simulink model "EnrouleurHG_Bode"  (R2024b)
settings: Solver=VariableStepAuto  StartTime=0.0  StopTime=1.2  RelTol=1e-3
values from neighbouring files (symbols this model uses):
  fv = 0    [parametres.m]
  Jm = 13.1/1000/10000    (= 1.31e-06)    [parametres.m]
  Kadapt = Kcapt/Rt    (= 52.1518917524)    [parametres.m]
  Kcapt = 8192/2/pi    (= 1303.79729381)    [parametres.m]
  Kcm = 25.5e-3    (= 0.0255)    [parametres.m]
  KCou_I = 900    [parametres.m]
  KCou_P = 2000    [parametres.m]
  KDSI = KPos_D*80/1000000    (= 0.0736)    [parametres.m]
  Kem = 1/(374 *2*pi/60)    (= 0.0255328785709)    [parametres.m]
  KPos_I = 270    [parametres.m]
  KPos_P = 215    [parametres.m]
  KPSI = KPos_P*10/1000    (= 2.15)    [parametres.m]
  Lm = 0.77e-3    (= 0.00077)    [parametres.m]
  r = 1/18    (= 0.0555555555556)    [parametres.m]
  Rm = 7.36    [parametres.m]
  Rt = 25    [parametres.m]
libraries: simulink x2, slctrl_linear x1
settings Model: Creator=xavier.pessoles2  LastModifiedBy=xpess

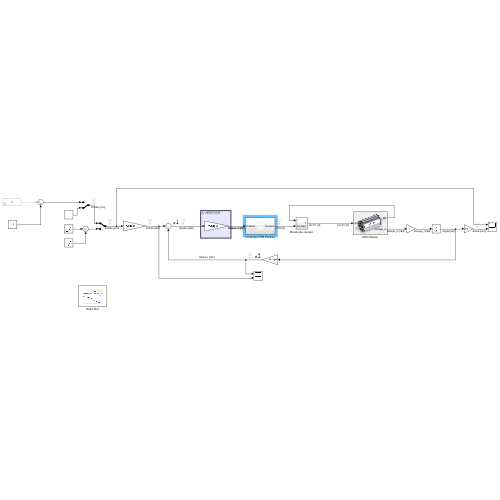
[thumbnail: Simulink's stored preview of the top-level diagram]
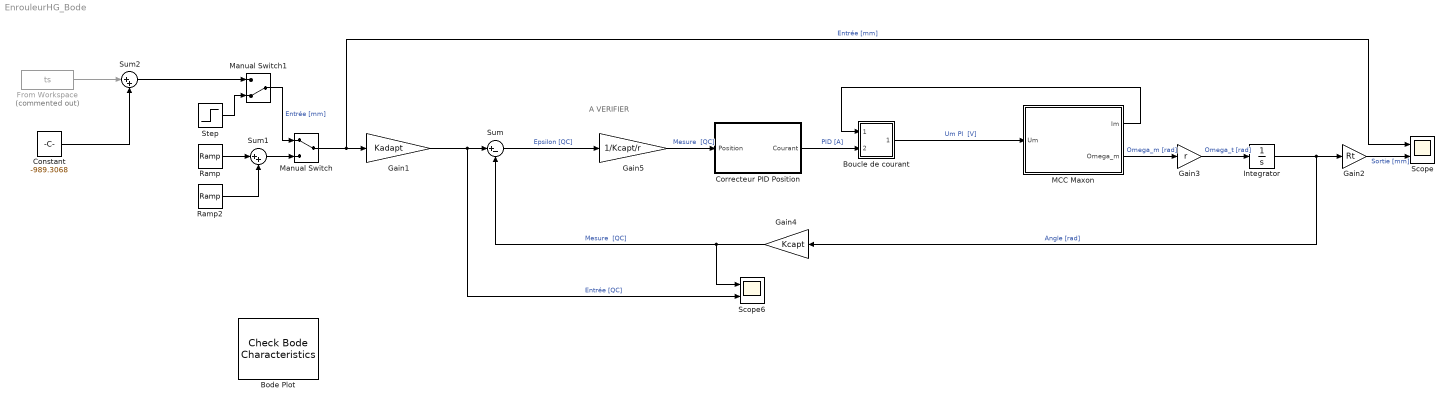
== system EnrouleurHG_Bode ==
  note: A VERIFIER
  Bode Plot : slctrl_linear/Check Bode  Characteristics  InstantiateOnLoad=on  SaveOperatingPoints=off  LinearizationIOs={'/Sum', 1, 'in', 'on', '';'/Gain4', 1, 'out', 'on', ''}  LinearizeAt=SnapshotTimes  SnapshotTimes=[0]  TriggerType=rising  SampleTime=auto  RateConversionMethod=zoh  PreWarpFreq=10  UseExactDelayModel=off  UseFullBlockNameLabels=off  UseBusSignalLabels=off  enabled=on  stopWhenAssertionFail=off  export=off  ViewDlgPos=[1 49 1280 599.333333333333]  OpenViewOnLoad=off  LaunchViewOnOpen=on  FrequencyUnits=rad/s  MagnitudeUnits=dB  PhaseUnits=deg  TimeUnits=seconds  EnableUpperBound=off  UpperBoundFrequencies=[]  UpperBoundMagnitudes=[]  EnableLowerBound=off  LowerBoundFrequencies=[]  LowerBoundMagnitudes=[]
      settings: LibrarySourceBlock=slctrlblks/Linear Analysis Plots/Bode Plot  SaveToWorkspace=off  SaveName=sys
  Boucle de courant : Subsystem
  Constant : Constant  Value=-989.3068
  Correcteur PID Position : Subsystem
  From Workspace : FromWorkspace  Commented=on  VariableName=ts
  Gain1 : Gain  Gain=Kadapt
  Gain2 : Gain  Gain=Rt
  Gain3 : Gain  Gain=r
  Gain4 : Gain  Gain=Kcapt
  Gain5 : Gain  Gain=1/Kcapt/r
  Integrator : Integrator
  MCC Maxon : Subsystem
      mask Display: image('MCC.png');
  Manual Switch : ManualSwitch
  Manual Switch1 : ManualSwitch  CurrentSetting=0
  Ramp : simulink/Sources/Ramp  slope=378  start=0  InitialOutput=0
  Ramp2 : simulink/Sources/Ramp  slope=-378  start=1  InitialOutput=0
  Scope : Scope  NumInputPorts=2
  Scope6 : Scope  NumInputPorts=2
  Step : Step  Time=0  After=0  SampleTime=0
  Sum : Sum  Inputs=|+-
  Sum1 : Sum  Inputs=|++
  Sum2 : Sum  Inputs=|++
  wires:
  Gain3/1 -> Integrator/1  "Omega_t [rad]"
  MCC Maxon/2(Omega_m) -> Gain3/1  "Omega_m [rad]"
  Sum/1 -> Gain5/1  "Epsilon [QC]"
  MCC Maxon/1(Im) -> Boucle de courant/1(In1)
  Boucle de courant/1(Out1) -> MCC Maxon/1(Um)  "Um PI  [V]"
  Gain4/1 -> Scope6/1, Sum/2  "Mesure  [QC]"
  Gain1/1 -> Sum/1, Scope6/2  "Entrée [QC]"
  Gain2/1 -> Scope/2  "Sortie [mm]"
  Integrator/1 -> Gain2/1, Gain4/1  "Angle [rad]"
  Ramp/1 -> Sum1/1
  Ramp2/1 -> Sum1/2
  Sum1/1 -> Manual Switch/2
  Manual Switch/1 -> Gain1/1, Scope/1  "Entrée [mm]"
  Gain5/1 -> Correcteur PID Position/1(Position)  "Mesure  [QC]"
  Manual Switch1/1 -> Manual Switch/1  "Entrée [mm]"
  Step/1 -> Manual Switch1/2
  From Workspace/1 -> Sum2/1
  Sum2/1 -> Manual Switch1/1
  Constant/1 -> Sum2/2
  Correcteur PID Position/1(Courant) -> Boucle de courant/2(Courant)  "PID [A]"

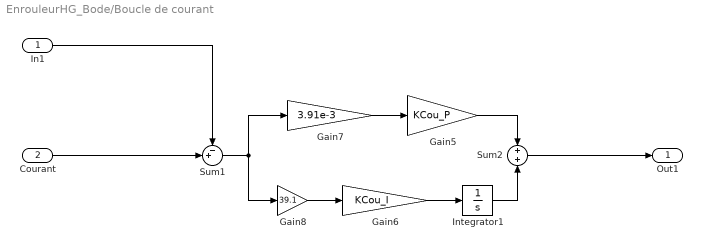
== system EnrouleurHG_Bode/Boucle de courant ==
  In1 : Inport
  Courant : Inport  Port=2
  Gain5 : Gain  Gain=KCou_P
  Gain6 : Gain  Gain=KCou_I
  Gain7 : Gain  Gain=3.91e-3
  Gain8 : Gain  Gain=39.1
  Integrator1 : Integrator
  Sum1 : Sum  Inputs=-+|
  Sum2 : Sum  Inputs=+|+
  Out1 : Outport
  wires:
  Sum1/1 -> Gain7/1, Gain8/1
  Gain5/1 -> Sum2/1
  Sum2/1 -> Out1/1
  Integrator1/1 -> Sum2/2
  Gain8/1 -> Gain6/1
  In1/1 -> Sum1/1
  Gain7/1 -> Gain5/1
  Gain6/1 -> Integrator1/1
  Courant/1 -> Sum1/2

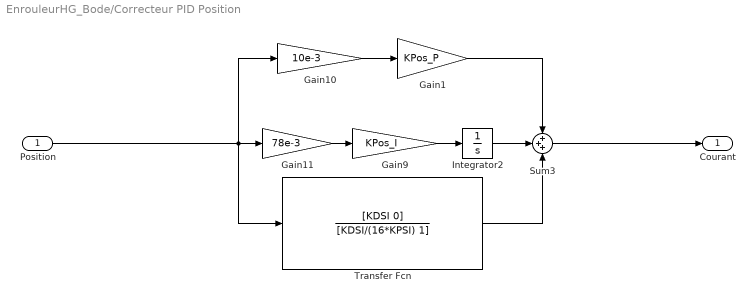
== system EnrouleurHG_Bode/Correcteur PID Position ==
  Position : Inport
  Gain1 : Gain  Gain=KPos_P
  Gain10 : Gain  Gain=10e-3
  Gain11 : Gain  Gain=78e-3
  Gain9 : Gain  Gain=KPos_I
  Integrator2 : Integrator
  Sum3 : Sum  Inputs=+++
  Transfer Fcn : TransferFcn  Numerator=[KDSI 0]  Denominator=[KDSI/(16*KPSI) 1]
  Courant : Outport
  wires:
  Gain1/1 -> Sum3/1
  Position/1 -> Gain10/1, Transfer Fcn/1, Gain11/1
  Gain9/1 -> Integrator2/1
  Sum3/1 -> Courant/1
  Integrator2/1 -> Sum3/2
  Gain10/1 -> Gain1/1
  Gain11/1 -> Gain9/1
  Transfer Fcn/1 -> Sum3/3

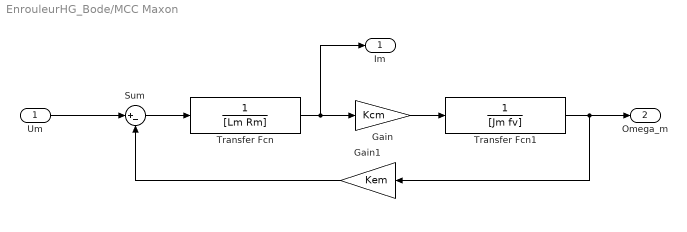
== system EnrouleurHG_Bode/MCC Maxon ==
  Um : Inport
  Gain : Gain  Gain=Kcm
  Gain1 : Gain  Gain=Kem
  Sum : Sum  Inputs=|+-
  Transfer Fcn : TransferFcn  Denominator=[Lm Rm]
  Transfer Fcn1 : TransferFcn  Denominator=[Jm fv]
  Im : Outport
  Omega_m : Outport  Port=2
  wires:
  Transfer Fcn/1 -> Im/1, Gain/1
  Transfer Fcn1/1 -> Omega_m/1, Gain1/1
  Gain/1 -> Transfer Fcn1/1
  Gain1/1 -> Sum/2
  Um/1 -> Sum/1
  Sum/1 -> Transfer Fcn/1
